simulink model "ASM_Traffic_V2X_Complete_Model_2"  (R2019a)
settings: Solver=ode1  StartTime=SIM.tstart.v  StopTime=Inf  FixedStep=SIM.StepSize.v  RelTol=1e-3
PostLoadFcn:
  | if any(exist('dsrtsu_mdlpostloadfcn', 'file') ~= 0), dsrtsu_mdlpostloadfcn('Execute', bdroot); end
  | try, asm_mdl_postloadfcn(bdroot, 'UpdateModel', 2200); catch, disp(lasterr); end,
undefined symbols (not defined in the file): _SensorPnts_1, _SensorPnts_13, _SensorPnts_17, _SensorPnts_21, _SensorPnts_25, _SensorPnts_29, _SensorPnts_33, _SensorPnts_37, _SensorPnts_41, _SensorPnts_45, _SensorPnts_49, _SensorPnts_5, _SensorPnts_53, _SensorPnts_57, _SensorPnts_9, _to_, CPT, G5A, ITS, MDL, rad, s_to_rpm, SIM
libraries: simulink x169, ASM_VehicleDynamics_lib x126, ASM_Traffic_lib x83, ASM_Utils_lib x49, mdbs x45, ASM_Environment_lib x17, dspindex x12, dsaV2xLibraryAux x10, dsmpblib x6, dsaV2xAsn1Library x4, dsaV2xLibrary x4, ASM_BrakeHydraulics_lib x4
(part 15 of 36)

== system ASM_Traffic_V2X_Complete_Model_2/MDLUserInterface/Environment/MDL_PAR/Fellow_VehicleLights ==
  Bus Creator2 : BusCreator  Inputs=15
  Fellow10_VehicleLights : Subsystem
  Fellow11_VehicleLights : Subsystem
  Fellow12_VehicleLights : Subsystem
  Fellow13_VehicleLights : Subsystem
  Fellow14_VehicleLights : Subsystem
  Fellow15_VehicleLights : Subsystem
  Fellow1_VehicleLights : Subsystem
  Fellow2_VehicleLights : Subsystem
  Fellow3_VehicleLights : Subsystem
  Fellow4_VehicleLights : Subsystem
  Fellow5_VehicleLights : Subsystem
  Fellow6_VehicleLights : Subsystem
  Fellow7_VehicleLights : Subsystem
  Fellow8_VehicleLights : Subsystem
  Fellow9_VehicleLights : Subsystem
  Terminator : Terminator
  tag scope: TAG_SW_FellowVehicleLights_Signals=global
  wires:
  [TAG_SW_FellowVehicleLights_Signals] -> Terminator/1
  Fellow1_VehicleLights/1(Out1) -> Bus Creator2/1  "Fellow1_VehicleLights"
  Fellow2_VehicleLights/1(Out1) -> Bus Creator2/2  "Fellow2_VehicleLights"
  Bus Creator2/1 -> [TAG_SW_FellowVehicleLights_Signals]
  Fellow3_VehicleLights/1(Out1) -> Bus Creator2/3  "Fellow3_VehicleLights"
  Fellow4_VehicleLights/1(Out1) -> Bus Creator2/4  "Fellow4_VehicleLights"
  Fellow5_VehicleLights/1(Out1) -> Bus Creator2/5  "Fellow5_VehicleLights"
  Fellow6_VehicleLights/1(Out1) -> Bus Creator2/6  "Fellow6_VehicleLights"
  Fellow7_VehicleLights/1(Out1) -> Bus Creator2/7  "Fellow7_VehicleLights"
  Fellow8_VehicleLights/1(Out1) -> Bus Creator2/8  "Fellow8_VehicleLights"
  Fellow9_VehicleLights/1(Out1) -> Bus Creator2/9  "Fellow9_VehicleLights"
  Fellow10_VehicleLights/1(Out1) -> Bus Creator2/10  "Fellow10_VehicleLights"
  Fellow11_VehicleLights/1(Out1) -> Bus Creator2/11  "Fellow11_VehicleLights"
  Fellow12_VehicleLights/1(Out1) -> Bus Creator2/12  "Fellow12_VehicleLights"
  Fellow13_VehicleLights/1(Out1) -> Bus Creator2/13  "Fellow13_VehicleLights"
  Fellow14_VehicleLights/1(Out1) -> Bus Creator2/14  "Fellow14_VehicleLights"
  Fellow15_VehicleLights/1(Out1) -> Bus Creator2/15  "Fellow15_VehicleLights"

== system ASM_Traffic_V2X_Complete_Model_2/MDLUserInterface/Environment/MDL_PAR/ManeuverControl ==
  Enable_ManeuverStart : Subsystem
      mask Display: disp('Enable ManeuverStart')
  MANEUVER_START : ASM_Utils_lib/ModelDeskInterface/ManeuverControl/MANEUVER_START  Tag=ASM_SUBCOMPONENT  MDLDCtrl_ManeuverStart=0  ASMProperties=struct('Name','MANEUVER_START','Version','2.0','Library','ASM_Utils_lib')  ASMInstanceName=maneuver_start  ASMInstanceID=1
  MANEUVER_STOP : ASM_Utils_lib/ModelDeskInterface/ManeuverControl/MANEUVER_STOP  Tag=ASM_SUBCOMPONENT  MDLDCtrl_ManeuverStop=0  ASMProperties=struct('Name','MANEUVER_STOP','Version','2.0','Library','ASM_Utils_lib')  ASMInstanceName=maneuver_stop  ASMInstanceID=1
  Mux1 : Mux
  RESET : ASM_Utils_lib/ModelDeskInterface/ManeuverControl/RESET  Tag=ASM_SUBCOMPONENT  MDLDCtrl_Reset=0  ASMProperties=struct('Name','RESET','Version','2.0','Library','ASM_Utils_lib')  ASMInstanceName=reset  ASMInstanceID=1
  Sw_ManualDriving[1ManSched|2Manual] : Constant
  Sw_StartManeuverAtSimStart[0|1] : Constant
  tag scope: TAG_Sw_ManeuverControl=global
  wires:
  MANEUVER_START/1 -> Enable_ManeuverStart/2(In)
  Enable_ManeuverStart/1(Out) -> Mux1/1
  Sw_StartManeuverAtSimStart[0|1]/1 -> Enable_ManeuverStart/1(Sw_StartManeuverAtSimStart[0|1])
  RESET/1 -> Mux1/4
  MANEUVER_STOP/1 -> Mux1/2
  Mux1/1 -> [TAG_Sw_ManeuverControl]
  Sw_ManualDriving[1ManSched|2Manual]/1 -> Mux1/3

== system ASM_Traffic_V2X_Complete_Model_2/MDLUserInterface/Environment/MDL_PAR/ManeuverSettings ==
  Bus Creator2 : BusCreator  Inputs=7
  Pos_BrakePedal_Seg_BrakeUntilStop[%] : Constant  Value=15
  Pos_BrakePedal_Seg_Standstill[%] : Constant  Value=15
  Pos_BrakePedal_State_Brake[%] : Constant  Value=15
  Pos_BrakePedal_State_Wait[%] : Constant  Value=70
  Pos_ClutchPedal_Seg_Standstill[%] : Constant  Value=0
  Rate_Angle_SteeringWheel_State_Wait[deg|s] : Constant  Value=360
  RelOffset_z_Init_Reset_Manual[m] : Constant  Value=0.01
  tag scope: TAG_Sw_ManeuverSettings=global
  wires:
  Pos_ClutchPedal_Seg_Standstill[%]/1 -> Bus Creator2/5  "Pos_ClutchPedal_Seg_Standstill[%]"
  Pos_BrakePedal_Seg_Standstill[%]/1 -> Bus Creator2/4  "Pos_BrakePedal_Seg_Standstill[%]"
  Pos_BrakePedal_Seg_BrakeUntilStop[%]/1 -> Bus Creator2/3  "Pos_BrakePedal_Seg_BrakeUntilStop[%]"
  Pos_BrakePedal_State_Wait[%]/1 -> Bus Creator2/2  "Pos_BrakePedal_State_Wait[%]"
  Pos_BrakePedal_State_Brake[%]/1 -> Bus Creator2/1  "Pos_BrakePedal_State_Brake[%]"
  Rate_Angle_SteeringWheel_State_Wait[deg|s]/1 -> Bus Creator2/6  "Rate_Angle_SteeringWheel_State_Wait[deg|s]"
  Bus Creator2/1 -> [TAG_Sw_ManeuverSettings]
  RelOffset_z_Init_Reset_Manual[m]/1 -> Bus Creator2/7  "RelOffset_z_Init_Reset_Manual[m]"

== system ASM_Traffic_V2X_Complete_Model_2/MDLUserInterface/Environment/MDL_PAR/ManualControl ==
  Angle_SteeringWheel[deg] : Constant  Value=0
  Bus Creator : BusCreator  Inputs=10
  Bus Creator1 : BusCreator  Inputs=3
  Bus Creator2 : BusCreator  Inputs=3
  Gear[] : Constant  Value=0
  LaneIdx_Ref[] : Constant  Value=0
  Pos_AccPedal[%] : Constant  Value=0
  Pos_BrakePedal[%] : Constant  Value=0
  Pos_ClutchPedal[%] : Constant  Value=100
  SW_BrakeLight[0Off|1On] : Constant  Value=0
  SW_ManualControl_Lights[1Maneuver|2Manual] : Constant
  SW_ParkingBrake[0Off|1On] : Constant  Value=0
  SW_TipTronic[-1Down|0Off|1Up] : Constant  Value=0
  SW_TurnLights[0Off|1Left|2Right|3Both] : Constant  Value=0
  SelectorLever[] : Constant  Value=0
  SelectorLever_Mode[1Stim|2Driver] : Constant  Value=2
  Sw_StartButton[0Off|1On] : Constant  Value=0
  Sw_StartButton_Mode[1Manual|2ManSched] : Constant
  Sw_Starter_Mode[1Stim|2PermanentOn] : Constant  Value=2
  Terminator : Terminator
  Trq_Steering[Nm] : Constant  Value=0
  d_Ref[m] : Constant  Value=0
  v_Vehicle_Ref[m|s] : Constant  Value=0
  tag scope: TAG_Const_PedalsManualDriving=global, TAG_SW_ASMVehicleLights_Signals=global, TAG_SW_ParkingBrake=global, TAG_SW_SelectorLever_Mode=global, TAG_SW_TipShift=global, TAG_StartButton_Signals=global
  wires:
  Pos_BrakePedal[%]/1 -> Bus Creator/2  "Pos_BrakePedal[%]"
  Angle_SteeringWheel[deg]/1 -> Bus Creator/5  "Angle_SteeringWheel[deg]"
  v_Vehicle_Ref[m|s]/1 -> Bus Creator/6  "v_Vehicle_Ref[m|s]"
  Gear[]/1 -> Bus Creator/4  "Gear[]"
  Pos_ClutchPedal[%]/1 -> Bus Creator/3  "Pos_ClutchPedal[%]"
  Pos_AccPedal[%]/1 -> Bus Creator/1  "Pos_AccPedal[%]"
  d_Ref[m]/1 -> Bus Creator/7  "d_Ref[m]"
  LaneIdx_Ref[]/1 -> Bus Creator/8  "LaneIdx_Ref[]"
  Bus Creator/1 -> [TAG_Const_PedalsManualDriving]
  SW_TipTronic[-1Down|0Off|1Up]/1 -> [TAG_SW_TipShift]
  SW_ParkingBrake[0Off|1On]/1 -> [TAG_SW_ParkingBrake]
  SW_BrakeLight[0Off|1On]/1 -> Bus Creator1/2  "SW_BrakeLight[0Off|1On]"
  SW_TurnLights[0Off|1Left|2Right|3Both]/1 -> Bus Creator1/3  "SW_TurnLights[0Off|1Left|2Right|3Both]"
  Bus Creator1/1 -> [TAG_SW_ASMVehicleLights_Signals]
  [TAG_SW_ASMVehicleLights_Signals] -> Terminator/1
  SW_ManualControl_Lights[1Maneuver|2Manual]/1 -> Bus Creator1/1  "SW_ManualControl_Lights[1Maneuver|2Manual]"
  Trq_Steering[Nm]/1 -> Bus Creator/9  "Trq_Steering[Nm]"
  SelectorLever[]/1 -> Bus Creator/10  "SelectorLever[]"
  SelectorLever_Mode[1Stim|2Driver]/1 -> [TAG_SW_SelectorLever_Mode]
  Sw_Starter_Mode[1Stim|2PermanentOn]/1 -> Bus Creator2/3  "Sw_Starter_Mode[1Stim|2PermanentOn]"
  Sw_StartButton[0Off|1On]/1 -> Bus Creator2/1  "Sw_StartButton[0Off|1On]"
  Bus Creator2/1 -> [TAG_StartButton_Signals]
  Sw_StartButton_Mode[1Manual|2ManSched]/1 -> Bus Creator2/2  "Sw_StartButton_Mode[1Manual|2ManSched]"

== system ASM_Traffic_V2X_Complete_Model_2/MDLUserInterface/Environment/MDL_PAR/Objects_DataStreams ==
  Bus Creator : BusCreator  Inputs=8
  Bus Creator1 : BusCreator  Inputs=1
  DataStream_1 : Subsystem
  DataStream_2 : Subsystem
  DataStream_3 : Subsystem
  DataStream_4 : Subsystem
  DataStream_5 : Subsystem
  DataStream_6 : Subsystem
  DataStream_7 : Subsystem
  DataStream_8 : Subsystem
  Terminator : Terminator
  tag scope: TAG_Objects_DataStreams=global
  wires:
  DataStream_8/1(DataStream_8[]) -> Bus Creator/8  "DataStream_8[]"
  DataStream_7/1(DataStream_7[]) -> Bus Creator/7  "DataStream_7[]"
  DataStream_6/1(DataStream_6[]) -> Bus Creator/6  "DataStream_6[]"
  DataStream_5/1(DataStream_5[]) -> Bus Creator/5  "DataStream_5[]"
  DataStream_4/1(DataStream_4[]) -> Bus Creator/4  "DataStream_4[]"
  DataStream_3/1(DataStream_3[]) -> Bus Creator/3  "DataStream_3[]"
  DataStream_2/1(DataStream_2[]) -> Bus Creator/2  "DataStream_2[]"
  DataStream_1/1(DataStream_1[]) -> Bus Creator/1  "DataStream_1[]"
  [TAG_Objects_DataStreams] -> Terminator/1
  [ASMBUS_Environment_Maneuver] -> DataStream_8/1(Maneuver_Signals[]), DataStream_7/1(Maneuver_Signals[]), DataStream_6/1(Maneuver_Signals[]), DataStream_5/1(Maneuver_Signals[])
  Bus Creator/1 -> Bus Creator1/1  "Objects_DataStreams[]"
  Bus Creator1/1 -> [TAG_Objects_DataStreams]

== system ASM_Traffic_V2X_Complete_Model_2/MDLUserInterface/Environment/MDL_PAR/SimulationControl ==
  note: 0 : Do not keep vehicle position at any condition.
      | 1 : Keep vehicle position at special conditions, e.g. if roll/pitch angle exceeds limits (prevents vehicle from falling over).
  Max_Angle_Pitch[deg] : Constant  Value=89
  Max_Angle_Roll[deg] : Constant  Value=89
  Mux : Mux  Inputs=2
  Sw_Keep_VehiclePosition[0Off|1On] : Constant
  tag scope: Tag_MaxAngleRollPitch=global, Tag_Sw_Keep_VehiclePosition=global
  wires:
  Sw_Keep_VehiclePosition[0Off|1On]/1 -> [Tag_Sw_Keep_VehiclePosition]
  Mux/1 -> [Tag_MaxAngleRollPitch]
  Max_Angle_Pitch[deg]/1 -> Mux/2
  Max_Angle_Roll[deg]/1 -> Mux/1

== system ASM_Traffic_V2X_Complete_Model_2/MDLUserInterface/Environment/MDL_PAR/Testbench ==
  Sw_Testbench[0|1] : Constant  Value=0
  n_Engine_Testbench[rpm] : Constant  Value=1000
  tag scope: TAG_SW_Testbench=global, TAG_n_Engine_Set=global
  wires:
  Sw_Testbench[0|1]/1 -> [TAG_SW_Testbench]
  n_Engine_Testbench[rpm]/1 -> [TAG_n_Engine_Set]

== system ASM_Traffic_V2X_Complete_Model_2/MDLUserInterface/Environment/MDL_PAR/TrafficControl ==
  Sw_TrafficEnable[0Off|1On] : Constant
  tag scope: TAG_Sw_TrafficEnable=global
  wires:
  Sw_TrafficEnable[0Off|1On]/1 -> [TAG_Sw_TrafficEnable]

== system ASM_Traffic_V2X_Complete_Model_2/MDLUserInterface/Environment/MDL_PAR/Vehicle_Inits ==
  Mux : Mux  Inputs=6
  v_x_Init[km|h] : Constant  Value=0  VectorParams1D=off
  v_y_Init[m|s] : Constant  Value=0  VectorParams1D=off
  v_z_Init[m|s] : Constant  Value=0  VectorParams1D=off
  w_x_Init[rad|s] : Constant  Value=0  VectorParams1D=off
  w_y_Init[rad|s] : Constant  Value=0  VectorParams1D=off
  w_z_Init[rad|s] : Constant  Value=0  VectorParams1D=off
  tag scope: TAG_Vehicle_Init=global
  wires:
  Mux/1 -> [TAG_Vehicle_Init]
  v_x_Init[km|h]/1 -> Mux/1  "v_x_Init[km|h]"
  w_x_Init[rad|s]/1 -> Mux/4  "w_x_Init[rad|s]"
  w_y_Init[rad|s]/1 -> Mux/5  "w_y_Init[rad|s]"
  w_z_Init[rad|s]/1 -> Mux/6  "w_z_Init[rad|s]"
  v_z_Init[m|s]/1 -> Mux/3  "v_z_Init[km|h]"
  v_y_Init[m|s]/1 -> Mux/2  "v_y_Init[km|h]"

== system ASM_Traffic_V2X_Complete_Model_2/MDLUserInterface/ModelDesk_Plotting/ModelDesk_PlotSignalCollector/InfoBlock ==

== system ASM_Traffic_V2X_Complete_Model_2/MDLUserInterface/MotionDeskInterface/Fellow_VehicleLights/Fellow1 ==
  SW_Signals_UserInterface : Inport
  v_fellow[m|s] : Inport  Port=2
  TurnLights[0|1|2|3] : Inport  Port=3
  Acceleration[m|s2] : simulink/Discrete/Discrete Derivative  gainval=1.0  ICPrevScaledInput=0.0  OutMin=[]  OutMax=[]  OutDataType=fixdt(1, 16)  OutScaling=2^-10  DoSatur=off
  Bus Selector : BusSelector  OutputSignals=SW_ManualControl_Lights[1Scheduler|2Manual],SW_BrakeLight[0Off|1On],SW_TurnLights[0Off|1Left|2Right|3Both]
  Compare_Both : simulink/Logic and Bit Operations/Compare To Constant  relop===  const=3  OutDataTypeStr=boolean
  Compare_Brakelight : simulink/Logic and Bit Operations/Compare To Constant  relop=<  const=-0.2  OutDataTypeStr=boolean
  Compare_Turnlight_L : simulink/Logic and Bit Operations/Compare To Constant  relop===  const=1  OutDataTypeStr=boolean
  Compare_Turnlight_R : simulink/Logic and Bit Operations/Compare To Constant  relop===  const=2  OutDataTypeStr=boolean
  Data Type Conversion1 : DataTypeConversion  OutDataTypeStr=boolean
  Data Type Conversion2 : DataTypeConversion  OutDataTypeStr=uint32
  Data Type Conversion3 : DataTypeConversion  OutDataTypeStr=uint32
  Data Type Conversion4 : DataTypeConversion  OutDataTypeStr=uint32
  Logical Operator : Logic  Operator=OR  AllPortsSameDT=off  OutDataTypeStr=boolean
  Logical Operator1 : Logic  Operator=OR  AllPortsSameDT=off  OutDataTypeStr=boolean
  Multiport Switch : MultiPortSwitch  Inputs=2
  Multiport Switch4 : MultiPortSwitch  Inputs=2
  Mux16 : Mux  Inputs=3
  FellowLights : Outport
  wires:
  Data Type Conversion4/1 -> Multiport Switch4/2
  Data Type Conversion2/1 -> Multiport Switch4/3
  Data Type Conversion1/1 -> Multiport Switch/3
  Data Type Conversion3/1 -> Multiport Switch4/1, Multiport Switch/1
  SW_Signals_UserInterface/1 -> Bus Selector/1
  Acceleration[m|s2]/1 -> Compare_Brakelight/1
  Mux16/1 -> FellowLights/1
  TurnLights[0|1|2|3]/1 -> Data Type Conversion4/1
  v_fellow[m|s]/1 -> Acceleration[m|s2]/1
  Bus Selector/3 -> Data Type Conversion2/1  "<SW_TurnLights[0Off|1Left|2Right|3Both]>"
  Multiport Switch4/1 -> Compare_Both/1, Compare_Turnlight_R/1, Compare_Turnlight_L/1
  Logical Operator1/1 -> Mux16/3
  Logical Operator/1 -> Mux16/2
  Compare_Both/1 -> Logical Operator/2, Logical Operator1/2
  Compare_Turnlight_R/1 -> Logical Operator1/1
  Compare_Turnlight_L/1 -> Logical Operator/1
  Multiport Switch/1 -> Mux16/1
  Bus Selector/2 -> Data Type Conversion1/1  "<SW_BrakeLight[0Off|1On]>"
  Compare_Brakelight/1 -> Multiport Switch/2
  Bus Selector/1 -> Data Type Conversion3/1  "<SW_ManualControl_Lights[1Scheduler|2Manual]>"

== system ASM_Traffic_V2X_Complete_Model_2/MDLUserInterface/MotionDeskInterface/Fellow_VehicleLights/Fellow10 ==
  SW_Signals_UserInterface : Inport
  v_fellow[m|s] : Inport  Port=2
  TurnLights[0|1|2|3] : Inport  Port=3
  Acceleration[m|s2] : simulink/Discrete/Discrete Derivative  gainval=1.0  ICPrevScaledInput=0.0  OutMin=[]  OutMax=[]  OutDataType=fixdt(1, 16)  OutScaling=2^-10  DoSatur=off
  Bus Selector : BusSelector  OutputSignals=SW_ManualControl_Lights[1Scheduler|2Manual],SW_BrakeLight[0Off|1On],SW_TurnLights[0Off|1Left|2Right|3Both]
  Compare_Both : simulink/Logic and Bit Operations/Compare To Constant  relop===  const=3  OutDataTypeStr=boolean
  Compare_Brakelight : simulink/Logic and Bit Operations/Compare To Constant  relop=<  const=-0.2  OutDataTypeStr=boolean
  Compare_Turnlight_L : simulink/Logic and Bit Operations/Compare To Constant  relop===  const=1  OutDataTypeStr=boolean
  Compare_Turnlight_R : simulink/Logic and Bit Operations/Compare To Constant  relop===  const=2  OutDataTypeStr=boolean
  Data Type Conversion1 : DataTypeConversion  OutDataTypeStr=boolean
  Data Type Conversion2 : DataTypeConversion  OutDataTypeStr=uint32
  Data Type Conversion3 : DataTypeConversion  OutDataTypeStr=uint32
  Data Type Conversion4 : DataTypeConversion  OutDataTypeStr=uint32
  Logical Operator : Logic  Operator=OR  AllPortsSameDT=off  OutDataTypeStr=boolean
  Logical Operator1 : Logic  Operator=OR  AllPortsSameDT=off  OutDataTypeStr=boolean
  Multiport Switch : MultiPortSwitch  Inputs=2
  Multiport Switch4 : MultiPortSwitch  Inputs=2
  Mux16 : Mux  Inputs=3
  FellowLights : Outport
  wires:
  Bus Selector/1 -> Data Type Conversion3/1  "<SW_ManualControl_Lights[1Scheduler|2Manual]>"
  Compare_Brakelight/1 -> Multiport Switch/2
  Bus Selector/2 -> Data Type Conversion1/1  "<SW_BrakeLight[0Off|1On]>"
  Multiport Switch/1 -> Mux16/1
  Compare_Turnlight_L/1 -> Logical Operator/1
  Compare_Turnlight_R/1 -> Logical Operator1/1
  Compare_Both/1 -> Logical Operator1/2, Logical Operator/2
  Logical Operator/1 -> Mux16/2
  Logical Operator1/1 -> Mux16/3
  Multiport Switch4/1 -> Compare_Turnlight_L/1, Compare_Turnlight_R/1, Compare_Both/1
  Bus Selector/3 -> Data Type Conversion2/1  "<SW_TurnLights[0Off|1Left|2Right|3Both]>"
  v_fellow[m|s]/1 -> Acceleration[m|s2]/1
  TurnLights[0|1|2|3]/1 -> Data Type Conversion4/1
  Mux16/1 -> FellowLights/1
  Acceleration[m|s2]/1 -> Compare_Brakelight/1
  SW_Signals_UserInterface/1 -> Bus Selector/1
  Data Type Conversion3/1 -> Multiport Switch/1, Multiport Switch4/1
  Data Type Conversion1/1 -> Multiport Switch/3
  Data Type Conversion2/1 -> Multiport Switch4/3
  Data Type Conversion4/1 -> Multiport Switch4/2

== system ASM_Traffic_V2X_Complete_Model_2/MDLUserInterface/MotionDeskInterface/Fellow_VehicleLights/Fellow11 ==
  SW_Signals_UserInterface : Inport
  v_fellow[m|s] : Inport  Port=2
  TurnLights[0|1|2|3] : Inport  Port=3
  Acceleration[m|s2] : simulink/Discrete/Discrete Derivative  gainval=1.0  ICPrevScaledInput=0.0  OutMin=[]  OutMax=[]  OutDataType=fixdt(1, 16)  OutScaling=2^-10  DoSatur=off
  Bus Selector : BusSelector  OutputSignals=SW_ManualControl_Lights[1Scheduler|2Manual],SW_BrakeLight[0Off|1On],SW_TurnLights[0Off|1Left|2Right|3Both]
  Compare_Both : simulink/Logic and Bit Operations/Compare To Constant  relop===  const=3  OutDataTypeStr=boolean
  Compare_Brakelight : simulink/Logic and Bit Operations/Compare To Constant  relop=<  const=-0.2  OutDataTypeStr=boolean
  Compare_Turnlight_L : simulink/Logic and Bit Operations/Compare To Constant  relop===  const=1  OutDataTypeStr=boolean
  Compare_Turnlight_R : simulink/Logic and Bit Operations/Compare To Constant  relop===  const=2  OutDataTypeStr=boolean
  Data Type Conversion1 : DataTypeConversion  OutDataTypeStr=boolean
  Data Type Conversion2 : DataTypeConversion  OutDataTypeStr=uint32
  Data Type Conversion3 : DataTypeConversion  OutDataTypeStr=uint32
  Data Type Conversion4 : DataTypeConversion  OutDataTypeStr=uint32
  Logical Operator : Logic  Operator=OR  AllPortsSameDT=off  OutDataTypeStr=boolean
  Logical Operator1 : Logic  Operator=OR  AllPortsSameDT=off  OutDataTypeStr=boolean
  Multiport Switch : MultiPortSwitch  Inputs=2
  Multiport Switch4 : MultiPortSwitch  Inputs=2
  Mux16 : Mux  Inputs=3
  FellowLights : Outport
  wires:
  Data Type Conversion4/1 -> Multiport Switch4/2
  Data Type Conversion2/1 -> Multiport Switch4/3
  Data Type Conversion1/1 -> Multiport Switch/3
  Data Type Conversion3/1 -> Multiport Switch4/1, Multiport Switch/1
  SW_Signals_UserInterface/1 -> Bus Selector/1
  Acceleration[m|s2]/1 -> Compare_Brakelight/1
  Mux16/1 -> FellowLights/1
  TurnLights[0|1|2|3]/1 -> Data Type Conversion4/1
  v_fellow[m|s]/1 -> Acceleration[m|s2]/1
  Bus Selector/3 -> Data Type Conversion2/1  "<SW_TurnLights[0Off|1Left|2Right|3Both]>"
  Multiport Switch4/1 -> Compare_Both/1, Compare_Turnlight_R/1, Compare_Turnlight_L/1
  Logical Operator1/1 -> Mux16/3
  Logical Operator/1 -> Mux16/2
  Compare_Both/1 -> Logical Operator/2, Logical Operator1/2
  Compare_Turnlight_R/1 -> Logical Operator1/1
  Compare_Turnlight_L/1 -> Logical Operator/1
  Multiport Switch/1 -> Mux16/1
  Bus Selector/2 -> Data Type Conversion1/1  "<SW_BrakeLight[0Off|1On]>"
  Compare_Brakelight/1 -> Multiport Switch/2
  Bus Selector/1 -> Data Type Conversion3/1  "<SW_ManualControl_Lights[1Scheduler|2Manual]>"

== system ASM_Traffic_V2X_Complete_Model_2/MDLUserInterface/MotionDeskInterface/Fellow_VehicleLights/Fellow12 ==
  SW_Signals_UserInterface : Inport
  v_fellow[m|s] : Inport  Port=2
  TurnLights[0|1|2|3] : Inport  Port=3
  Acceleration[m|s2] : simulink/Discrete/Discrete Derivative  gainval=1.0  ICPrevScaledInput=0.0  OutMin=[]  OutMax=[]  OutDataType=fixdt(1, 16)  OutScaling=2^-10  DoSatur=off
  Bus Selector : BusSelector  OutputSignals=SW_ManualControl_Lights[1Scheduler|2Manual],SW_BrakeLight[0Off|1On],SW_TurnLights[0Off|1Left|2Right|3Both]
  Compare_Both : simulink/Logic and Bit Operations/Compare To Constant  relop===  const=3  OutDataTypeStr=boolean
  Compare_Brakelight : simulink/Logic and Bit Operations/Compare To Constant  relop=<  const=-0.2  OutDataTypeStr=boolean
  Compare_Turnlight_L : simulink/Logic and Bit Operations/Compare To Constant  relop===  const=1  OutDataTypeStr=boolean
  Compare_Turnlight_R : simulink/Logic and Bit Operations/Compare To Constant  relop===  const=2  OutDataTypeStr=boolean
  Data Type Conversion1 : DataTypeConversion  OutDataTypeStr=boolean
  Data Type Conversion2 : DataTypeConversion  OutDataTypeStr=uint32
  Data Type Conversion3 : DataTypeConversion  OutDataTypeStr=uint32
  Data Type Conversion4 : DataTypeConversion  OutDataTypeStr=uint32
  Logical Operator : Logic  Operator=OR  AllPortsSameDT=off  OutDataTypeStr=boolean
  Logical Operator1 : Logic  Operator=OR  AllPortsSameDT=off  OutDataTypeStr=boolean
  Multiport Switch : MultiPortSwitch  Inputs=2
  Multiport Switch4 : MultiPortSwitch  Inputs=2
  Mux16 : Mux  Inputs=3
  FellowLights : Outport
  wires:
  Bus Selector/1 -> Data Type Conversion3/1  "<SW_ManualControl_Lights[1Scheduler|2Manual]>"
  Compare_Brakelight/1 -> Multiport Switch/2
  Bus Selector/2 -> Data Type Conversion1/1  "<SW_BrakeLight[0Off|1On]>"
  Multiport Switch/1 -> Mux16/1
  Compare_Turnlight_L/1 -> Logical Operator/1
  Compare_Turnlight_R/1 -> Logical Operator1/1
  Compare_Both/1 -> Logical Operator1/2, Logical Operator/2
  Logical Operator/1 -> Mux16/2
  Logical Operator1/1 -> Mux16/3
  Multiport Switch4/1 -> Compare_Turnlight_L/1, Compare_Turnlight_R/1, Compare_Both/1
  Bus Selector/3 -> Data Type Conversion2/1  "<SW_TurnLights[0Off|1Left|2Right|3Both]>"
  v_fellow[m|s]/1 -> Acceleration[m|s2]/1
  TurnLights[0|1|2|3]/1 -> Data Type Conversion4/1
  Mux16/1 -> FellowLights/1
  Acceleration[m|s2]/1 -> Compare_Brakelight/1
  SW_Signals_UserInterface/1 -> Bus Selector/1
  Data Type Conversion3/1 -> Multiport Switch/1, Multiport Switch4/1
  Data Type Conversion1/1 -> Multiport Switch/3
  Data Type Conversion2/1 -> Multiport Switch4/3
  Data Type Conversion4/1 -> Multiport Switch4/2

== system ASM_Traffic_V2X_Complete_Model_2/MDLUserInterface/MotionDeskInterface/Fellow_VehicleLights/Fellow13 ==
  SW_Signals_UserInterface : Inport
  v_fellow[m|s] : Inport  Port=2
  TurnLights[0|1|2|3] : Inport  Port=3
  Acceleration[m|s2] : simulink/Discrete/Discrete Derivative  gainval=1.0  ICPrevScaledInput=0.0  OutMin=[]  OutMax=[]  OutDataType=fixdt(1, 16)  OutScaling=2^-10  DoSatur=off
  Bus Selector : BusSelector  OutputSignals=SW_ManualControl_Lights[1Scheduler|2Manual],SW_BrakeLight[0Off|1On],SW_TurnLights[0Off|1Left|2Right|3Both]
  Compare_Both : simulink/Logic and Bit Operations/Compare To Constant  relop===  const=3  OutDataTypeStr=boolean
  Compare_Brakelight : simulink/Logic and Bit Operations/Compare To Constant  relop=<  const=-0.2  OutDataTypeStr=boolean
  Compare_Turnlight_L : simulink/Logic and Bit Operations/Compare To Constant  relop===  const=1  OutDataTypeStr=boolean
  Compare_Turnlight_R : simulink/Logic and Bit Operations/Compare To Constant  relop===  const=2  OutDataTypeStr=boolean
  Data Type Conversion1 : DataTypeConversion  OutDataTypeStr=boolean
  Data Type Conversion2 : DataTypeConversion  OutDataTypeStr=uint32
  Data Type Conversion3 : DataTypeConversion  OutDataTypeStr=uint32
  Data Type Conversion4 : DataTypeConversion  OutDataTypeStr=uint32
  Logical Operator : Logic  Operator=OR  AllPortsSameDT=off  OutDataTypeStr=boolean
  Logical Operator1 : Logic  Operator=OR  AllPortsSameDT=off  OutDataTypeStr=boolean
  Multiport Switch : MultiPortSwitch  Inputs=2
  Multiport Switch4 : MultiPortSwitch  Inputs=2
  Mux16 : Mux  Inputs=3
  FellowLights : Outport
  wires:
  Data Type Conversion4/1 -> Multiport Switch4/2
  Data Type Conversion2/1 -> Multiport Switch4/3
  Data Type Conversion1/1 -> Multiport Switch/3
  Data Type Conversion3/1 -> Multiport Switch4/1, Multiport Switch/1
  SW_Signals_UserInterface/1 -> Bus Selector/1
  Acceleration[m|s2]/1 -> Compare_Brakelight/1
  Mux16/1 -> FellowLights/1
  TurnLights[0|1|2|3]/1 -> Data Type Conversion4/1
  v_fellow[m|s]/1 -> Acceleration[m|s2]/1
  Bus Selector/3 -> Data Type Conversion2/1  "<SW_TurnLights[0Off|1Left|2Right|3Both]>"
  Multiport Switch4/1 -> Compare_Both/1, Compare_Turnlight_R/1, Compare_Turnlight_L/1
  Logical Operator1/1 -> Mux16/3
  Logical Operator/1 -> Mux16/2
  Compare_Both/1 -> Logical Operator/2, Logical Operator1/2
  Compare_Turnlight_R/1 -> Logical Operator1/1
  Compare_Turnlight_L/1 -> Logical Operator/1
  Multiport Switch/1 -> Mux16/1
  Bus Selector/2 -> Data Type Conversion1/1  "<SW_BrakeLight[0Off|1On]>"
  Compare_Brakelight/1 -> Multiport Switch/2
  Bus Selector/1 -> Data Type Conversion3/1  "<SW_ManualControl_Lights[1Scheduler|2Manual]>"

== system ASM_Traffic_V2X_Complete_Model_2/MDLUserInterface/MotionDeskInterface/Fellow_VehicleLights/Fellow14 ==
  SW_Signals_UserInterface : Inport
  v_fellow[m|s] : Inport  Port=2
  TurnLights[0|1|2|3] : Inport  Port=3
  Acceleration[m|s2] : simulink/Discrete/Discrete Derivative  gainval=1.0  ICPrevScaledInput=0.0  OutMin=[]  OutMax=[]  OutDataType=fixdt(1, 16)  OutScaling=2^-10  DoSatur=off
  Bus Selector : BusSelector  OutputSignals=SW_ManualControl_Lights[1Scheduler|2Manual],SW_BrakeLight[0Off|1On],SW_TurnLights[0Off|1Left|2Right|3Both]
  Compare_Both : simulink/Logic and Bit Operations/Compare To Constant  relop===  const=3  OutDataTypeStr=boolean
  Compare_Brakelight : simulink/Logic and Bit Operations/Compare To Constant  relop=<  const=-0.2  OutDataTypeStr=boolean
  Compare_Turnlight_L : simulink/Logic and Bit Operations/Compare To Constant  relop===  const=1  OutDataTypeStr=boolean
  Compare_Turnlight_R : simulink/Logic and Bit Operations/Compare To Constant  relop===  const=2  OutDataTypeStr=boolean
  Data Type Conversion1 : DataTypeConversion  OutDataTypeStr=boolean
  Data Type Conversion2 : DataTypeConversion  OutDataTypeStr=uint32
  Data Type Conversion3 : DataTypeConversion  OutDataTypeStr=uint32
  Data Type Conversion4 : DataTypeConversion  OutDataTypeStr=uint32
  Logical Operator : Logic  Operator=OR  AllPortsSameDT=off  OutDataTypeStr=boolean
  Logical Operator1 : Logic  Operator=OR  AllPortsSameDT=off  OutDataTypeStr=boolean
  Multiport Switch : MultiPortSwitch  Inputs=2
  Multiport Switch4 : MultiPortSwitch  Inputs=2
  Mux16 : Mux  Inputs=3
  FellowLights : Outport
  wires:
  Bus Selector/1 -> Data Type Conversion3/1  "<SW_ManualControl_Lights[1Scheduler|2Manual]>"
  Compare_Brakelight/1 -> Multiport Switch/2
  Bus Selector/2 -> Data Type Conversion1/1  "<SW_BrakeLight[0Off|1On]>"
  Multiport Switch/1 -> Mux16/1
  Compare_Turnlight_L/1 -> Logical Operator/1
  Compare_Turnlight_R/1 -> Logical Operator1/1
  Compare_Both/1 -> Logical Operator1/2, Logical Operator/2
  Logical Operator/1 -> Mux16/2
  Logical Operator1/1 -> Mux16/3
  Multiport Switch4/1 -> Compare_Turnlight_L/1, Compare_Turnlight_R/1, Compare_Both/1
  Bus Selector/3 -> Data Type Conversion2/1  "<SW_TurnLights[0Off|1Left|2Right|3Both]>"
  v_fellow[m|s]/1 -> Acceleration[m|s2]/1
  TurnLights[0|1|2|3]/1 -> Data Type Conversion4/1
  Mux16/1 -> FellowLights/1
  Acceleration[m|s2]/1 -> Compare_Brakelight/1
  SW_Signals_UserInterface/1 -> Bus Selector/1
  Data Type Conversion3/1 -> Multiport Switch/1, Multiport Switch4/1
  Data Type Conversion1/1 -> Multiport Switch/3
  Data Type Conversion2/1 -> Multiport Switch4/3
  Data Type Conversion4/1 -> Multiport Switch4/2

== system ASM_Traffic_V2X_Complete_Model_2/MDLUserInterface/MotionDeskInterface/Fellow_VehicleLights/Fellow15 ==
  SW_Signals_UserInterface : Inport
  v_fellow[m|s] : Inport  Port=2
  TurnLights[0|1|2|3] : Inport  Port=3
  Acceleration[m|s2] : simulink/Discrete/Discrete Derivative  gainval=1.0  ICPrevScaledInput=0.0  OutMin=[]  OutMax=[]  OutDataType=fixdt(1, 16)  OutScaling=2^-10  DoSatur=off
  Bus Selector : BusSelector  OutputSignals=SW_ManualControl_Lights[1Scheduler|2Manual],SW_BrakeLight[0Off|1On],SW_TurnLights[0Off|1Left|2Right|3Both]
  Compare_Both : simulink/Logic and Bit Operations/Compare To Constant  relop===  const=3  OutDataTypeStr=boolean
  Compare_Brakelight : simulink/Logic and Bit Operations/Compare To Constant  relop=<  const=-0.2  OutDataTypeStr=boolean
  Compare_Turnlight_L : simulink/Logic and Bit Operations/Compare To Constant  relop===  const=1  OutDataTypeStr=boolean
  Compare_Turnlight_R : simulink/Logic and Bit Operations/Compare To Constant  relop===  const=2  OutDataTypeStr=boolean
  Data Type Conversion1 : DataTypeConversion  OutDataTypeStr=boolean
  Data Type Conversion2 : DataTypeConversion  OutDataTypeStr=uint32
  Data Type Conversion3 : DataTypeConversion  OutDataTypeStr=uint32
  Data Type Conversion4 : DataTypeConversion  OutDataTypeStr=uint32
  Logical Operator : Logic  Operator=OR  AllPortsSameDT=off  OutDataTypeStr=boolean
  Logical Operator1 : Logic  Operator=OR  AllPortsSameDT=off  OutDataTypeStr=boolean
  Multiport Switch : MultiPortSwitch  Inputs=2
  Multiport Switch4 : MultiPortSwitch  Inputs=2
  Mux16 : Mux  Inputs=3
  FellowLights : Outport
  wires:
  Data Type Conversion4/1 -> Multiport Switch4/2
  Data Type Conversion2/1 -> Multiport Switch4/3
  Data Type Conversion1/1 -> Multiport Switch/3
  Data Type Conversion3/1 -> Multiport Switch4/1, Multiport Switch/1
  SW_Signals_UserInterface/1 -> Bus Selector/1
  Acceleration[m|s2]/1 -> Compare_Brakelight/1
  Mux16/1 -> FellowLights/1
  TurnLights[0|1|2|3]/1 -> Data Type Conversion4/1
  v_fellow[m|s]/1 -> Acceleration[m|s2]/1
  Bus Selector/3 -> Data Type Conversion2/1  "<SW_TurnLights[0Off|1Left|2Right|3Both]>"
  Multiport Switch4/1 -> Compare_Both/1, Compare_Turnlight_R/1, Compare_Turnlight_L/1
  Logical Operator1/1 -> Mux16/3
  Logical Operator/1 -> Mux16/2
  Compare_Both/1 -> Logical Operator/2, Logical Operator1/2
  Compare_Turnlight_R/1 -> Logical Operator1/1
  Compare_Turnlight_L/1 -> Logical Operator/1
  Multiport Switch/1 -> Mux16/1
  Bus Selector/2 -> Data Type Conversion1/1  "<SW_BrakeLight[0Off|1On]>"
  Compare_Brakelight/1 -> Multiport Switch/2
  Bus Selector/1 -> Data Type Conversion3/1  "<SW_ManualControl_Lights[1Scheduler|2Manual]>"

== system ASM_Traffic_V2X_Complete_Model_2/MDLUserInterface/MotionDeskInterface/Fellow_VehicleLights/Fellow2 ==
  SW_Signals_UserInterface : Inport
  v_fellow[m|s] : Inport  Port=2
  TurnLights[0|1|2|3] : Inport  Port=3
  Acceleration[m|s2] : simulink/Discrete/Discrete Derivative  gainval=1.0  ICPrevScaledInput=0.0  OutMin=[]  OutMax=[]  OutDataType=fixdt(1, 16)  OutScaling=2^-10  DoSatur=off
  Bus Selector : BusSelector  OutputSignals=SW_ManualControl_Lights[1Scheduler|2Manual],SW_BrakeLight[0Off|1On],SW_TurnLights[0Off|1Left|2Right|3Both]
  Compare_Both : simulink/Logic and Bit Operations/Compare To Constant  relop===  const=3  OutDataTypeStr=boolean
  Compare_Brakelight : simulink/Logic and Bit Operations/Compare To Constant  relop=<  const=-0.2  OutDataTypeStr=boolean
  Compare_Turnlight_L : simulink/Logic and Bit Operations/Compare To Constant  relop===  const=1  OutDataTypeStr=boolean
  Compare_Turnlight_R : simulink/Logic and Bit Operations/Compare To Constant  relop===  const=2  OutDataTypeStr=boolean
  Data Type Conversion1 : DataTypeConversion  OutDataTypeStr=boolean
  Data Type Conversion2 : DataTypeConversion  OutDataTypeStr=uint32
  Data Type Conversion3 : DataTypeConversion  OutDataTypeStr=uint32
  Data Type Conversion4 : DataTypeConversion  OutDataTypeStr=uint32
  Logical Operator : Logic  Operator=OR  AllPortsSameDT=off  OutDataTypeStr=boolean
  Logical Operator1 : Logic  Operator=OR  AllPortsSameDT=off  OutDataTypeStr=boolean
  Multiport Switch : MultiPortSwitch  Inputs=2
  Multiport Switch4 : MultiPortSwitch  Inputs=2
  Mux16 : Mux  Inputs=3
  FellowLights : Outport
  wires:
  Bus Selector/1 -> Data Type Conversion3/1  "<SW_ManualControl_Lights[1Scheduler|2Manual]>"
  Compare_Brakelight/1 -> Multiport Switch/2
  Bus Selector/2 -> Data Type Conversion1/1  "<SW_BrakeLight[0Off|1On]>"
  Multiport Switch/1 -> Mux16/1
  Compare_Turnlight_L/1 -> Logical Operator/1
  Compare_Turnlight_R/1 -> Logical Operator1/1
  Compare_Both/1 -> Logical Operator1/2, Logical Operator/2
  Logical Operator/1 -> Mux16/2
  Logical Operator1/1 -> Mux16/3
  Multiport Switch4/1 -> Compare_Turnlight_L/1, Compare_Turnlight_R/1, Compare_Both/1
  Bus Selector/3 -> Data Type Conversion2/1  "<SW_TurnLights[0Off|1Left|2Right|3Both]>"
  v_fellow[m|s]/1 -> Acceleration[m|s2]/1
  TurnLights[0|1|2|3]/1 -> Data Type Conversion4/1
  Mux16/1 -> FellowLights/1
  Acceleration[m|s2]/1 -> Compare_Brakelight/1
  SW_Signals_UserInterface/1 -> Bus Selector/1
  Data Type Conversion3/1 -> Multiport Switch/1, Multiport Switch4/1
  Data Type Conversion1/1 -> Multiport Switch/3
  Data Type Conversion2/1 -> Multiport Switch4/3
  Data Type Conversion4/1 -> Multiport Switch4/2

== system ASM_Traffic_V2X_Complete_Model_2/MDLUserInterface/MotionDeskInterface/Fellow_VehicleLights/Fellow3 ==
  SW_Signals_UserInterface : Inport
  v_fellow[m|s] : Inport  Port=2
  TurnLights[0|1|2|3] : Inport  Port=3
  Acceleration[m|s2] : simulink/Discrete/Discrete Derivative  gainval=1.0  ICPrevScaledInput=0.0  OutMin=[]  OutMax=[]  OutDataType=fixdt(1, 16)  OutScaling=2^-10  DoSatur=off
  Bus Selector : BusSelector  OutputSignals=SW_ManualControl_Lights[1Scheduler|2Manual],SW_BrakeLight[0Off|1On],SW_TurnLights[0Off|1Left|2Right|3Both]
  Compare_Both : simulink/Logic and Bit Operations/Compare To Constant  relop===  const=3  OutDataTypeStr=boolean
  Compare_Brakelight : simulink/Logic and Bit Operations/Compare To Constant  relop=<  const=-0.2  OutDataTypeStr=boolean
  Compare_Turnlight_L : simulink/Logic and Bit Operations/Compare To Constant  relop===  const=1  OutDataTypeStr=boolean
  Compare_Turnlight_R : simulink/Logic and Bit Operations/Compare To Constant  relop===  const=2  OutDataTypeStr=boolean
  Data Type Conversion1 : DataTypeConversion  OutDataTypeStr=boolean
  Data Type Conversion2 : DataTypeConversion  OutDataTypeStr=uint32
  Data Type Conversion3 : DataTypeConversion  OutDataTypeStr=uint32
  Data Type Conversion4 : DataTypeConversion  OutDataTypeStr=uint32
  Logical Operator : Logic  Operator=OR  AllPortsSameDT=off  OutDataTypeStr=boolean
  Logical Operator1 : Logic  Operator=OR  AllPortsSameDT=off  OutDataTypeStr=boolean
  Multiport Switch : MultiPortSwitch  Inputs=2
  Multiport Switch4 : MultiPortSwitch  Inputs=2
  Mux16 : Mux  Inputs=3
  FellowLights : Outport
  wires:
  Data Type Conversion4/1 -> Multiport Switch4/2
  Data Type Conversion2/1 -> Multiport Switch4/3
  Data Type Conversion1/1 -> Multiport Switch/3
  Data Type Conversion3/1 -> Multiport Switch4/1, Multiport Switch/1
  SW_Signals_UserInterface/1 -> Bus Selector/1
  Acceleration[m|s2]/1 -> Compare_Brakelight/1
  Mux16/1 -> FellowLights/1
  TurnLights[0|1|2|3]/1 -> Data Type Conversion4/1
  v_fellow[m|s]/1 -> Acceleration[m|s2]/1
  Bus Selector/3 -> Data Type Conversion2/1  "<SW_TurnLights[0Off|1Left|2Right|3Both]>"
  Multiport Switch4/1 -> Compare_Both/1, Compare_Turnlight_R/1, Compare_Turnlight_L/1
  Logical Operator1/1 -> Mux16/3
  Logical Operator/1 -> Mux16/2
  Compare_Both/1 -> Logical Operator/2, Logical Operator1/2
  Compare_Turnlight_R/1 -> Logical Operator1/1
  Compare_Turnlight_L/1 -> Logical Operator/1
  Multiport Switch/1 -> Mux16/1
  Bus Selector/2 -> Data Type Conversion1/1  "<SW_BrakeLight[0Off|1On]>"
  Compare_Brakelight/1 -> Multiport Switch/2
  Bus Selector/1 -> Data Type Conversion3/1  "<SW_ManualControl_Lights[1Scheduler|2Manual]>"

== system ASM_Traffic_V2X_Complete_Model_2/MDLUserInterface/MotionDeskInterface/Fellow_VehicleLights/Fellow4 ==
  SW_Signals_UserInterface : Inport
  v_fellow[m|s] : Inport  Port=2
  TurnLights[0|1|2|3] : Inport  Port=3
  Acceleration[m|s2] : simulink/Discrete/Discrete Derivative  gainval=1.0  ICPrevScaledInput=0.0  OutMin=[]  OutMax=[]  OutDataType=fixdt(1, 16)  OutScaling=2^-10  DoSatur=off
  Bus Selector : BusSelector  OutputSignals=SW_ManualControl_Lights[1Scheduler|2Manual],SW_BrakeLight[0Off|1On],SW_TurnLights[0Off|1Left|2Right|3Both]
  Compare_Both : simulink/Logic and Bit Operations/Compare To Constant  relop===  const=3  OutDataTypeStr=boolean
  Compare_Brakelight : simulink/Logic and Bit Operations/Compare To Constant  relop=<  const=-0.2  OutDataTypeStr=boolean
  Compare_Turnlight_L : simulink/Logic and Bit Operations/Compare To Constant  relop===  const=1  OutDataTypeStr=boolean
  Compare_Turnlight_R : simulink/Logic and Bit Operations/Compare To Constant  relop===  const=2  OutDataTypeStr=boolean
  Data Type Conversion1 : DataTypeConversion  OutDataTypeStr=boolean
  Data Type Conversion2 : DataTypeConversion  OutDataTypeStr=uint32
  Data Type Conversion3 : DataTypeConversion  OutDataTypeStr=uint32
  Data Type Conversion4 : DataTypeConversion  OutDataTypeStr=uint32
  Logical Operator : Logic  Operator=OR  AllPortsSameDT=off  OutDataTypeStr=boolean
  Logical Operator1 : Logic  Operator=OR  AllPortsSameDT=off  OutDataTypeStr=boolean
  Multiport Switch : MultiPortSwitch  Inputs=2
  Multiport Switch4 : MultiPortSwitch  Inputs=2
  Mux16 : Mux  Inputs=3
  FellowLights : Outport
  wires:
  Bus Selector/1 -> Data Type Conversion3/1  "<SW_ManualControl_Lights[1Scheduler|2Manual]>"
  Compare_Brakelight/1 -> Multiport Switch/2
  Bus Selector/2 -> Data Type Conversion1/1  "<SW_BrakeLight[0Off|1On]>"
  Multiport Switch/1 -> Mux16/1
  Compare_Turnlight_L/1 -> Logical Operator/1
  Compare_Turnlight_R/1 -> Logical Operator1/1
  Compare_Both/1 -> Logical Operator1/2, Logical Operator/2
  Logical Operator/1 -> Mux16/2
  Logical Operator1/1 -> Mux16/3
  Multiport Switch4/1 -> Compare_Turnlight_L/1, Compare_Turnlight_R/1, Compare_Both/1
  Bus Selector/3 -> Data Type Conversion2/1  "<SW_TurnLights[0Off|1Left|2Right|3Both]>"
  v_fellow[m|s]/1 -> Acceleration[m|s2]/1
  TurnLights[0|1|2|3]/1 -> Data Type Conversion4/1
  Mux16/1 -> FellowLights/1
  Acceleration[m|s2]/1 -> Compare_Brakelight/1
  SW_Signals_UserInterface/1 -> Bus Selector/1
  Data Type Conversion3/1 -> Multiport Switch/1, Multiport Switch4/1
  Data Type Conversion1/1 -> Multiport Switch/3
  Data Type Conversion2/1 -> Multiport Switch4/3
  Data Type Conversion4/1 -> Multiport Switch4/2

== system ASM_Traffic_V2X_Complete_Model_2/MDLUserInterface/MotionDeskInterface/Fellow_VehicleLights/Fellow5 ==
  SW_Signals_UserInterface : Inport
  v_fellow[m|s] : Inport  Port=2
  TurnLights[0|1|2|3] : Inport  Port=3
  Acceleration[m|s2] : simulink/Discrete/Discrete Derivative  gainval=1.0  ICPrevScaledInput=0.0  OutMin=[]  OutMax=[]  OutDataType=fixdt(1, 16)  OutScaling=2^-10  DoSatur=off
  Bus Selector : BusSelector  OutputSignals=SW_ManualControl_Lights[1Scheduler|2Manual],SW_BrakeLight[0Off|1On],SW_TurnLights[0Off|1Left|2Right|3Both]
  Compare_Both : simulink/Logic and Bit Operations/Compare To Constant  relop===  const=3  OutDataTypeStr=boolean
  Compare_Brakelight : simulink/Logic and Bit Operations/Compare To Constant  relop=<  const=-0.2  OutDataTypeStr=boolean
  Compare_Turnlight_L : simulink/Logic and Bit Operations/Compare To Constant  relop===  const=1  OutDataTypeStr=boolean
  Compare_Turnlight_R : simulink/Logic and Bit Operations/Compare To Constant  relop===  const=2  OutDataTypeStr=boolean
  Data Type Conversion1 : DataTypeConversion  OutDataTypeStr=boolean
  Data Type Conversion2 : DataTypeConversion  OutDataTypeStr=uint32
  Data Type Conversion3 : DataTypeConversion  OutDataTypeStr=uint32
  Data Type Conversion4 : DataTypeConversion  OutDataTypeStr=uint32
  Logical Operator : Logic  Operator=OR  AllPortsSameDT=off  OutDataTypeStr=boolean
  Logical Operator1 : Logic  Operator=OR  AllPortsSameDT=off  OutDataTypeStr=boolean
  Multiport Switch : MultiPortSwitch  Inputs=2
  Multiport Switch4 : MultiPortSwitch  Inputs=2
  Mux16 : Mux  Inputs=3
  FellowLights : Outport
  wires:
  Data Type Conversion4/1 -> Multiport Switch4/2
  Data Type Conversion2/1 -> Multiport Switch4/3
  Data Type Conversion1/1 -> Multiport Switch/3
  Data Type Conversion3/1 -> Multiport Switch4/1, Multiport Switch/1
  SW_Signals_UserInterface/1 -> Bus Selector/1
  Acceleration[m|s2]/1 -> Compare_Brakelight/1
  Mux16/1 -> FellowLights/1
  TurnLights[0|1|2|3]/1 -> Data Type Conversion4/1
  v_fellow[m|s]/1 -> Acceleration[m|s2]/1
  Bus Selector/3 -> Data Type Conversion2/1  "<SW_TurnLights[0Off|1Left|2Right|3Both]>"
  Multiport Switch4/1 -> Compare_Both/1, Compare_Turnlight_R/1, Compare_Turnlight_L/1
  Logical Operator1/1 -> Mux16/3
  Logical Operator/1 -> Mux16/2
  Compare_Both/1 -> Logical Operator/2, Logical Operator1/2
  Compare_Turnlight_R/1 -> Logical Operator1/1
  Compare_Turnlight_L/1 -> Logical Operator/1
  Multiport Switch/1 -> Mux16/1
  Bus Selector/2 -> Data Type Conversion1/1  "<SW_BrakeLight[0Off|1On]>"
  Compare_Brakelight/1 -> Multiport Switch/2
  Bus Selector/1 -> Data Type Conversion3/1  "<SW_ManualControl_Lights[1Scheduler|2Manual]>"

== system ASM_Traffic_V2X_Complete_Model_2/MDLUserInterface/MotionDeskInterface/Fellow_VehicleLights/Fellow6 ==
  SW_Signals_UserInterface : Inport
  v_fellow[m|s] : Inport  Port=2
  TurnLights[0|1|2|3] : Inport  Port=3
  Acceleration[m|s2] : simulink/Discrete/Discrete Derivative  gainval=1.0  ICPrevScaledInput=0.0  OutMin=[]  OutMax=[]  OutDataType=fixdt(1, 16)  OutScaling=2^-10  DoSatur=off
  Bus Selector : BusSelector  OutputSignals=SW_ManualControl_Lights[1Scheduler|2Manual],SW_BrakeLight[0Off|1On],SW_TurnLights[0Off|1Left|2Right|3Both]
  Compare_Both : simulink/Logic and Bit Operations/Compare To Constant  relop===  const=3  OutDataTypeStr=boolean
  Compare_Brakelight : simulink/Logic and Bit Operations/Compare To Constant  relop=<  const=-0.2  OutDataTypeStr=boolean
  Compare_Turnlight_L : simulink/Logic and Bit Operations/Compare To Constant  relop===  const=1  OutDataTypeStr=boolean
  Compare_Turnlight_R : simulink/Logic and Bit Operations/Compare To Constant  relop===  const=2  OutDataTypeStr=boolean
  Data Type Conversion1 : DataTypeConversion  OutDataTypeStr=boolean
  Data Type Conversion2 : DataTypeConversion  OutDataTypeStr=uint32
  Data Type Conversion3 : DataTypeConversion  OutDataTypeStr=uint32
  Data Type Conversion4 : DataTypeConversion  OutDataTypeStr=uint32
  Logical Operator : Logic  Operator=OR  AllPortsSameDT=off  OutDataTypeStr=boolean
  Logical Operator1 : Logic  Operator=OR  AllPortsSameDT=off  OutDataTypeStr=boolean
  Multiport Switch : MultiPortSwitch  Inputs=2
  Multiport Switch4 : MultiPortSwitch  Inputs=2
  Mux16 : Mux  Inputs=3
  FellowLights : Outport
  wires:
  Bus Selector/1 -> Data Type Conversion3/1  "<SW_ManualControl_Lights[1Scheduler|2Manual]>"
  Compare_Brakelight/1 -> Multiport Switch/2
  Bus Selector/2 -> Data Type Conversion1/1  "<SW_BrakeLight[0Off|1On]>"
  Multiport Switch/1 -> Mux16/1
  Compare_Turnlight_L/1 -> Logical Operator/1
  Compare_Turnlight_R/1 -> Logical Operator1/1
  Compare_Both/1 -> Logical Operator1/2, Logical Operator/2
  Logical Operator/1 -> Mux16/2
  Logical Operator1/1 -> Mux16/3
  Multiport Switch4/1 -> Compare_Turnlight_L/1, Compare_Turnlight_R/1, Compare_Both/1
  Bus Selector/3 -> Data Type Conversion2/1  "<SW_TurnLights[0Off|1Left|2Right|3Both]>"
  v_fellow[m|s]/1 -> Acceleration[m|s2]/1
  TurnLights[0|1|2|3]/1 -> Data Type Conversion4/1
  Mux16/1 -> FellowLights/1
  Acceleration[m|s2]/1 -> Compare_Brakelight/1
  SW_Signals_UserInterface/1 -> Bus Selector/1
  Data Type Conversion3/1 -> Multiport Switch/1, Multiport Switch4/1
  Data Type Conversion1/1 -> Multiport Switch/3
  Data Type Conversion2/1 -> Multiport Switch4/3
  Data Type Conversion4/1 -> Multiport Switch4/2

== system ASM_Traffic_V2X_Complete_Model_2/MDLUserInterface/MotionDeskInterface/Fellow_VehicleLights/Fellow7 ==
  SW_Signals_UserInterface : Inport
  v_fellow[m|s] : Inport  Port=2
  TurnLights[0|1|2|3] : Inport  Port=3
  Acceleration[m|s2] : simulink/Discrete/Discrete Derivative  gainval=1.0  ICPrevScaledInput=0.0  OutMin=[]  OutMax=[]  OutDataType=fixdt(1, 16)  OutScaling=2^-10  DoSatur=off
  Bus Selector : BusSelector  OutputSignals=SW_ManualControl_Lights[1Scheduler|2Manual],SW_BrakeLight[0Off|1On],SW_TurnLights[0Off|1Left|2Right|3Both]
  Compare_Both : simulink/Logic and Bit Operations/Compare To Constant  relop===  const=3  OutDataTypeStr=boolean
  Compare_Brakelight : simulink/Logic and Bit Operations/Compare To Constant  relop=<  const=-0.2  OutDataTypeStr=boolean
  Compare_Turnlight_L : simulink/Logic and Bit Operations/Compare To Constant  relop===  const=1  OutDataTypeStr=boolean
  Compare_Turnlight_R : simulink/Logic and Bit Operations/Compare To Constant  relop===  const=2  OutDataTypeStr=boolean
  Data Type Conversion1 : DataTypeConversion  OutDataTypeStr=boolean
  Data Type Conversion2 : DataTypeConversion  OutDataTypeStr=uint32
  Data Type Conversion3 : DataTypeConversion  OutDataTypeStr=uint32
  Data Type Conversion4 : DataTypeConversion  OutDataTypeStr=uint32
  Logical Operator : Logic  Operator=OR  AllPortsSameDT=off  OutDataTypeStr=boolean
  Logical Operator1 : Logic  Operator=OR  AllPortsSameDT=off  OutDataTypeStr=boolean
  Multiport Switch : MultiPortSwitch  Inputs=2
  Multiport Switch4 : MultiPortSwitch  Inputs=2
  Mux16 : Mux  Inputs=3
  FellowLights : Outport
  wires:
  Data Type Conversion4/1 -> Multiport Switch4/2
  Data Type Conversion2/1 -> Multiport Switch4/3
  Data Type Conversion1/1 -> Multiport Switch/3
  Data Type Conversion3/1 -> Multiport Switch4/1, Multiport Switch/1
  SW_Signals_UserInterface/1 -> Bus Selector/1
  Acceleration[m|s2]/1 -> Compare_Brakelight/1
  Mux16/1 -> FellowLights/1
  TurnLights[0|1|2|3]/1 -> Data Type Conversion4/1
  v_fellow[m|s]/1 -> Acceleration[m|s2]/1
  Bus Selector/3 -> Data Type Conversion2/1  "<SW_TurnLights[0Off|1Left|2Right|3Both]>"
  Multiport Switch4/1 -> Compare_Both/1, Compare_Turnlight_R/1, Compare_Turnlight_L/1
  Logical Operator1/1 -> Mux16/3
  Logical Operator/1 -> Mux16/2
  Compare_Both/1 -> Logical Operator/2, Logical Operator1/2
  Compare_Turnlight_R/1 -> Logical Operator1/1
  Compare_Turnlight_L/1 -> Logical Operator/1
  Multiport Switch/1 -> Mux16/1
  Bus Selector/2 -> Data Type Conversion1/1  "<SW_BrakeLight[0Off|1On]>"
  Compare_Brakelight/1 -> Multiport Switch/2
  Bus Selector/1 -> Data Type Conversion3/1  "<SW_ManualControl_Lights[1Scheduler|2Manual]>"

== system ASM_Traffic_V2X_Complete_Model_2/MDLUserInterface/MotionDeskInterface/Fellow_VehicleLights/Fellow8 ==
  SW_Signals_UserInterface : Inport
  v_fellow[m|s] : Inport  Port=2
  TurnLights[0|1|2|3] : Inport  Port=3
  Acceleration[m|s2] : simulink/Discrete/Discrete Derivative  gainval=1.0  ICPrevScaledInput=0.0  OutMin=[]  OutMax=[]  OutDataType=fixdt(1, 16)  OutScaling=2^-10  DoSatur=off
  Bus Selector : BusSelector  OutputSignals=SW_ManualControl_Lights[1Scheduler|2Manual],SW_BrakeLight[0Off|1On],SW_TurnLights[0Off|1Left|2Right|3Both]
  Compare_Both : simulink/Logic and Bit Operations/Compare To Constant  relop===  const=3  OutDataTypeStr=boolean
  Compare_Brakelight : simulink/Logic and Bit Operations/Compare To Constant  relop=<  const=-0.2  OutDataTypeStr=boolean
  Compare_Turnlight_L : simulink/Logic and Bit Operations/Compare To Constant  relop===  const=1  OutDataTypeStr=boolean
  Compare_Turnlight_R : simulink/Logic and Bit Operations/Compare To Constant  relop===  const=2  OutDataTypeStr=boolean
  Data Type Conversion1 : DataTypeConversion  OutDataTypeStr=boolean
  Data Type Conversion2 : DataTypeConversion  OutDataTypeStr=uint32
  Data Type Conversion3 : DataTypeConversion  OutDataTypeStr=uint32
  Data Type Conversion4 : DataTypeConversion  OutDataTypeStr=uint32
  Logical Operator : Logic  Operator=OR  AllPortsSameDT=off  OutDataTypeStr=boolean
  Logical Operator1 : Logic  Operator=OR  AllPortsSameDT=off  OutDataTypeStr=boolean
  Multiport Switch : MultiPortSwitch  Inputs=2
  Multiport Switch4 : MultiPortSwitch  Inputs=2
  Mux16 : Mux  Inputs=3
  FellowLights : Outport
  wires:
  Bus Selector/1 -> Data Type Conversion3/1  "<SW_ManualControl_Lights[1Scheduler|2Manual]>"
  Compare_Brakelight/1 -> Multiport Switch/2
  Bus Selector/2 -> Data Type Conversion1/1  "<SW_BrakeLight[0Off|1On]>"
  Multiport Switch/1 -> Mux16/1
  Compare_Turnlight_L/1 -> Logical Operator/1
  Compare_Turnlight_R/1 -> Logical Operator1/1
  Compare_Both/1 -> Logical Operator1/2, Logical Operator/2
  Logical Operator/1 -> Mux16/2
  Logical Operator1/1 -> Mux16/3
  Multiport Switch4/1 -> Compare_Turnlight_L/1, Compare_Turnlight_R/1, Compare_Both/1
  Bus Selector/3 -> Data Type Conversion2/1  "<SW_TurnLights[0Off|1Left|2Right|3Both]>"
  v_fellow[m|s]/1 -> Acceleration[m|s2]/1
  TurnLights[0|1|2|3]/1 -> Data Type Conversion4/1
  Mux16/1 -> FellowLights/1
  Acceleration[m|s2]/1 -> Compare_Brakelight/1
  SW_Signals_UserInterface/1 -> Bus Selector/1
  Data Type Conversion3/1 -> Multiport Switch/1, Multiport Switch4/1
  Data Type Conversion1/1 -> Multiport Switch/3
  Data Type Conversion2/1 -> Multiport Switch4/3
  Data Type Conversion4/1 -> Multiport Switch4/2
